simulink model "rms_evaluation2"  (R2013b)
settings: Solver=FixedStepDiscrete  StartTime=0.0  StopTime=0.1  FixedStep=1e-5  RelTol=1e-3
settings Model: Creator=Abel  LastModifiedBy=Abel

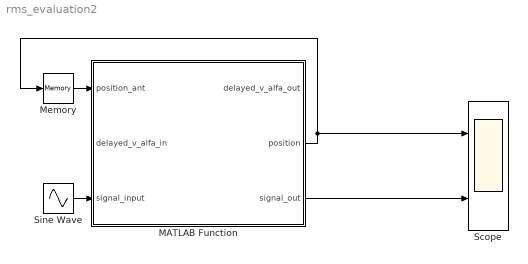
== system rms_evaluation2 ==
  MATLAB Function : MATLAB Function  TreatAsAtomicUnit=on
  Memory : Memory  X0=1  LinearizeAsDelay=on
  Scope : Scope  NumInputPorts=2
      settings: YMin=-5~-5  YMax=5~5
  Sine Wave : Sin  Frequency=2*pi*50  SampleTime=0
  wires:
  Memory/1 -> MATLAB Function/1(position_ant)
  MATLAB Function/2(position) -> Memory/1, Scope/1
  Sine Wave/1 -> MATLAB Function/3(signal_input)
  MATLAB Function/3(signal_out) -> Scope/2

== matlab function rms_evaluation2/MATLAB Function ==
  data: delayed_v_alfa_out output; position_ant input; delayed_v_alfa_in input; position output; signal_input input; signal_out output
function [delayed_v_alfa_out, position, signal_out]= fcn(position_ant, delayed_v_alfa_in, signal_input)
%#codegen

%position = (position>(SIZE_VECTOR-2)) ? 0 : position + 1;
position = position_ant;
signal_out = abs(signal_input);

if (position_ant > 199)
    position = 0;
else
    position = position_ant + 1;
end

%       Atraso de v_alfa
% 		signal_input = v_alfa;
% 		signal_output = delayed_v_alfa[position];
% 		delayed_v_alfa[position]  = signal_input;
% 		v_alfa_delayed = signal_output;

delayed_v_alfa_out = 0:0:200;


end
